simulink model "VSC"  (R2015b)
settings: Solver=VariableStepAuto  StartTime=0.0  StopTime=10.0  RelTol=1e-3
values from neighbouring files (symbols this model uses):
  T = 2    [matlab.mat]
undefined symbols (not defined in the file or in its folder): sys, sys_p
settings Model: Creator=Jcama  LastModifiedBy=Jcama

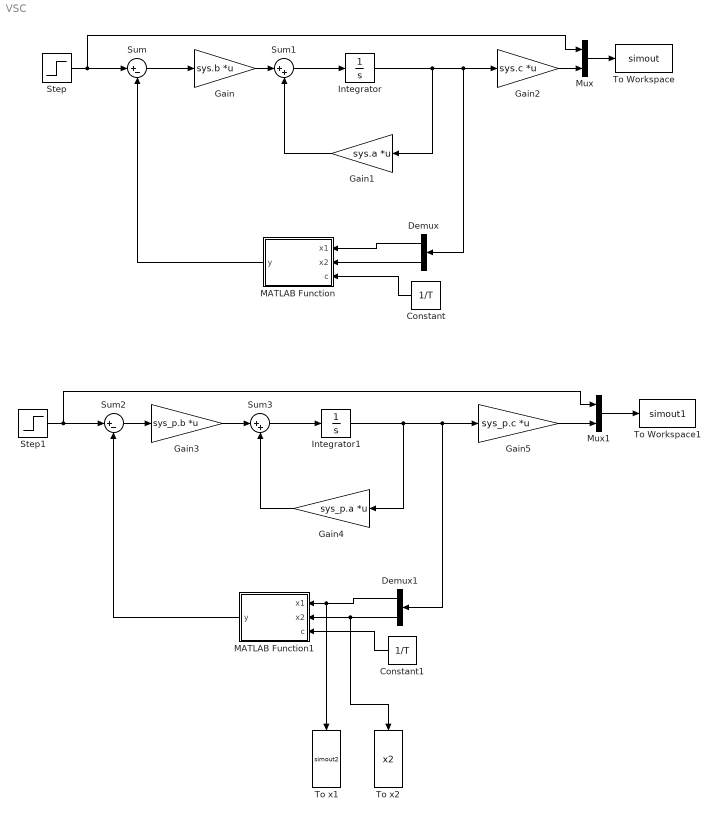
== system VSC ==
  Constant : Constant  Value=1/T
  Constant1 : Constant  Value=1/T
  Demux : Demux  Outputs=2
  Demux1 : Demux  Outputs=2
  Gain : Gain  Gain=sys.b  Multiplication=Matrix(K*u)
  Gain1 : Gain  Gain=sys.a  Multiplication=Matrix(K*u)
  Gain2 : Gain  Gain=sys.c  Multiplication=Matrix(K*u)
  Gain3 : Gain  Gain=sys_p.b  Multiplication=Matrix(K*u)
  Gain4 : Gain  Gain=sys_p.a  Multiplication=Matrix(K*u)
  Gain5 : Gain  Gain=sys_p.c  Multiplication=Matrix(K*u)
  Integrator : Integrator
  Integrator1 : Integrator
  MATLAB Function : MATLAB Function  TreatAsAtomicUnit=on
  MATLAB Function1 : MATLAB Function  TreatAsAtomicUnit=on
  Mux : Mux  Inputs=2
  Mux1 : Mux  Inputs=2
  Step : Step  Time=0  SampleTime=0
  Step1 : Step  Time=0  SampleTime=0
  Sum : Sum  Inputs=|+-
  Sum1 : Sum  Inputs=|++
  Sum2 : Sum  Inputs=|+-
  Sum3 : Sum  Inputs=|++
  To Workspace : ToWorkspace  VariableName=simout  SaveFormat=Timeseries  SampleTime=-1
  To Workspace1 : ToWorkspace  VariableName=simout1  SaveFormat=Timeseries  SampleTime=-1
  To x1 : ToWorkspace  VariableName=simout2  SaveFormat=Timeseries  SampleTime=-1
  To x2 : ToWorkspace  VariableName=x2  SaveFormat=Timeseries  SampleTime=-1
  wires:
  Integrator/1 -> Gain2/1, Demux/1, Gain1/1
  Step/1 -> Mux/1, Sum/1
  Sum/1 -> Gain/1
  Gain/1 -> Sum1/1
  Sum1/1 -> Integrator/1
  Gain1/1 -> Sum1/2
  Demux/1 -> MATLAB Function/1(x1)
  Demux/2 -> MATLAB Function/2(x2)
  Constant/1 -> MATLAB Function/3(c)
  MATLAB Function/1(y) -> Sum/2
  Gain2/1 -> Mux/2
  Mux/1 -> To Workspace/1
  Integrator1/1 -> Gain5/1, Demux1/1, Gain4/1
  Step1/1 -> Mux1/1, Sum2/1
  Sum2/1 -> Gain3/1
  Gain3/1 -> Sum3/1
  Sum3/1 -> Integrator1/1
  Gain4/1 -> Sum3/2
  Demux1/1 -> MATLAB Function1/1(x1), To x1/1
  Demux1/2 -> MATLAB Function1/2(x2), To x2/1
  Constant1/1 -> MATLAB Function1/3(c)
  MATLAB Function1/1(y) -> Sum2/2
  Gain5/1 -> Mux1/2
  Mux1/1 -> To Workspace1/1

== matlab function VSC/MATLAB Function1 ==
  data: x1 input; y output; x2 input; c input
function y = fcn(x1,x2,c)

Psi = ((c^2)/2 + 6*c - 10.01);
s = c * x1 + x2;
if (s * x1) > 0
    x1 = x1 * Psi;
else
    x1 = -x1 * Psi;
end

y = x1;

== matlab function VSC/MATLAB Function ==
  data: x1 input; y output; x2 input; c input
function y = fcn(x1,x2,c)

Psi = 12/c - 20.02 - 1/c^2;
s = c * x1 + x2;
if s * x2 > 0
    x2 = x2 * Psi;
else
    x2 = -x2 * Psi;
end

y = x2;
